simulink model "power_WITHOUT"  (Simulink 7.4)
settings: Solver=FixedStepDiscrete  SolverMode=SingleTasking  StartTime=0.0  StopTime=1  FixedStep=Ts  MaxStep=Ts*2  RelTol=1e-4  AbsTol=1e-4
PreLoadFcn:
  | Ts=50e-6;
undefined symbols (not defined in the file): D1, Delta
libraries: powerlib x9, powerlib_extras x1
Description:
  | Copyright 2008 The MathWorks(TM), Inc.
settings Model: Creator=hyp01  LastModifiedBy=Bharath  ExtModeTrigMode=oneshot  ExtModeArmWhenConnect=off  ExtModeAutoUpdateStatusClock=off
settings DataIOCC: LimitDataPoints=off  SaveFinalState=on  SaveFormat=StructureWithTime  SaveOutput=off  SaveTime=off  SignalLoggingName=sigsOut
settings OptimizationCC: BooleanDataType=off  InlineInvariantSignals=on  InitFltsAndDblsToZero=on  EfficientMapNaN2IntZero=off
settings DebuggingCC: CheckExecutionContextPreStartOutputMsg=on  CheckExecutionContextRuntimeOutputMsg=on  SignalResolutionControl=TryResolveAllWithWarning  SolverPrmCheckMsg=none  MultiTaskDSMMsg=warning  MultiTaskCondExecSysMsg=none  StrictBusMsg=None
settings HardwareCC: TargetUnknown=on
settings RTWCC: IncludeERTFirstTime=on

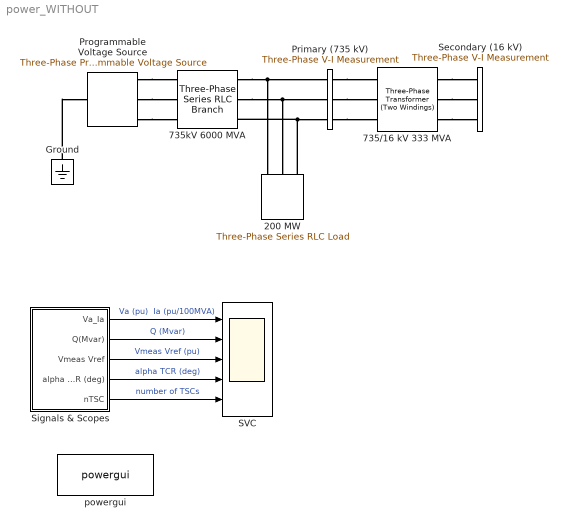
== system power_WITHOUT ==
  200 MW : powerlib/Elements/Three-Phase Series RLC Load  DialogController=POWERSYS.PowerSysDialog  PhysicalDomain=powersysdomain  SubClassName=unknown  LeftPortType=p1  RightPortType=p1  LConnTagsString=A|B|C  Configuration=Y (grounded)  NominalVoltage=735e3  NominalFrequency=60  ActivePower=200e6  InductivePower=0  CapacitivePower=0  Measurements=None
  735/16 kV 333 MVA : powerlib/Elements/Three-Phase Transformer (Two Windings)  DialogController=POWERSYS.PowerSysDialog  SystemSampleTime=-1  Winding1Connection=Yg  UNITS=pu  NominalPower=[333e6 , 60 ]  Winding1=[735e3 , 0.15/30/2 , 0.15*0.7]  Winding2Connection=Delta (D1)  Winding2=[ 16e3 , 0.15/30/2, 0.15*0.3]  SetSaturation=off  Rm=500  Lm=500  Saturation="[ 0,0  ;  0.005,1.2  ;  1.0,1.4 ]"  Hysteresis=off  DataFile='hysteresis'  SetInitialFlux=off  InitialFluxes=[ 0.8 , -0.8 , 0.7 ]  Measurements=None  MoreParameters=off  BreakLoop=off  DataType=off  TransfoNumber=0
  "735kV 6000 MVA " : powerlib/Elements/Three-Phase Series RLC Branch  DialogController=POWERSYS.PowerSysDialog  PhysicalDomain=powersysdomain  SubClassName=unknown  LeftPortType=p1  RightPortType=p1  LConnTagsString=A|B|C  RConnTagsString=A|B|C  BranchType=RL  Resistance=735e3^2/6000e6/10  Inductance=735e3^2/6000e6/(2*pi*60)  Capacitance=1.0  Measurements=None
  Ground : powerlib/Elements/Ground  DialogController=POWERSYS.PowerSysDialog  PhysicalDomain=powersysdomain  SubClassName=unknown  LeftPortType=p1  RightPortType=p1  LConnTagsString=a
  Primary (735 kV) : powerlib/Measurements/Three-Phase V-I Measurement  DialogController=POWERSYS.PowerSysDialog  SystemSampleTime=-1  VoltageMeasurement=phase-to-ground  SetLabelV=on  LabelV=Vabc_Prim  Vpu=on  CurrentMeasurement=yes  SetLabelI=on  LabelI=Iabc_Prim  Ipu=on  Pbase=100e6  Vbase=735e3  OutputType=Magnitude  PhasorSimulation=off  PSBequivalent=0
  Programmable Voltage Source : powerlib/Electrical Sources/Three-Phase Programmable Voltage Source  DialogController=POWERSYS.PowerSysDialog  SystemSampleTime=-1  PositiveSequence="[1.004*735e3 0  60]"  VariationEntity=Amplitude  VariationType=Table of time-amplitude pairs  VariationStep=-0.3  VariationRate=0.5  VariationMagnitude=0.4  VariationFrequency=2  VariationTiming=[0.1 1.2]  VariationPhaseA=off  Amplitudes=[1.0 1.025 0.93 1.0 ]  TimeValues=[0 0.1 0.4 0.7]  HarmonicGeneration=off  HarmonicA=[3 0.2 -25 0]  HarmonicB="[2 0.15  35 2]"  Timing="[0.1  0.6]"
  SVC : Scope  NumInputPorts=5
      settings: YMin=-1.5~-0.7~-1~-1~-1  YMax=1.5~-0.57~1~1~1  SaveName=VIabc_Prim  SampleInput=on  SampleTime=Ts
  Secondary (16 kV) : powerlib/Measurements/Three-Phase V-I Measurement  DialogController=POWERSYS.PowerSysDialog  SystemSampleTime=-1  VoltageMeasurement=phase-to-phase  SetLabelV=on  LabelV=Vabc_Sec  Vpu=on  CurrentMeasurement=no  SetLabelI=off  LabelI=Iabc_Sec  Ipu=off  Pbase=100e6  Vbase=16e3  OutputType=Magnitude  PhasorSimulation=off  PSBequivalent=0
  Signals & Scopes : Subsystem
  powergui : powerlib/powergui  Priority=2  SystemSampleTime=-1  SimulationMode=Discrete  SampleTime=Ts  frequency=60  SPID=off  DisableSnubberDevices=off  DisableRonSwitches=off  DisableVfSwitches=off  SwTol=0  Interpol=off  frequencyindice=60  echomessages=off  HookPort=off  DisplayEquations=off  FunctionMessages=off  EnableUseOfTLC=off  x0status=blocks  RestoreLinks=warning  Frange=[0:2:500]  Ylog=off  Xlog=on  ShowGrid=off  save=off  variable=ZData  ZoomFFT=on  StartTime=0.0  cycles=1  DisplayStyle=1  fundamental=60  FreqAxis=off  MaxFrequency=1000  frequencyindicesteady=1  RmsSteady=2  display=off  Ts=0  methode=off
  wires:
  Signals & Scopes/1(Va_Ia) -> SVC/1  "Va (pu)  Ia (pu/100MVA)"
  Signals & Scopes/3("Vmeas Vref ") -> SVC/3  "Vmeas Vref (pu)"
  Signals & Scopes/5(nTSC) -> SVC/5  "number of TSCs"
  Signals & Scopes/2(Q(Mvar)) -> SVC/2  "Q (Mvar)"
  Signals & Scopes/4(alpha TCR (deg)) -> SVC/4  "alpha TCR (deg)"
  connections:
  Ground/LConn1 -- Programmable Voltage Source/LConn1
  "735kV 6000 MVA "/RConn1 -- Primary (735 kV)/LConn1 -- 200 MW/LConn1
  "735kV 6000 MVA "/RConn2 -- Primary (735 kV)/LConn2 -- 200 MW/LConn2
  735/16 kV 333 MVA/RConn1 -- Secondary (16 kV)/LConn1
  735/16 kV 333 MVA/RConn3 -- Secondary (16 kV)/LConn3
  Programmable Voltage Source/RConn2 -- "735kV 6000 MVA "/LConn2
  Programmable Voltage Source/RConn3 -- "735kV 6000 MVA "/LConn3
  Programmable Voltage Source/RConn1 -- "735kV 6000 MVA "/LConn1
  735/16 kV 333 MVA/RConn2 -- Secondary (16 kV)/LConn2
  200 MW/LConn3 -- "735kV 6000 MVA "/RConn3 -- Primary (735 kV)/LConn3
  Primary (735 kV)/RConn1 -- 735/16 kV 333 MVA/LConn1
  Primary (735 kV)/RConn2 -- 735/16 kV 333 MVA/LConn2
  Primary (735 kV)/RConn3 -- 735/16 kV 333 MVA/LConn3

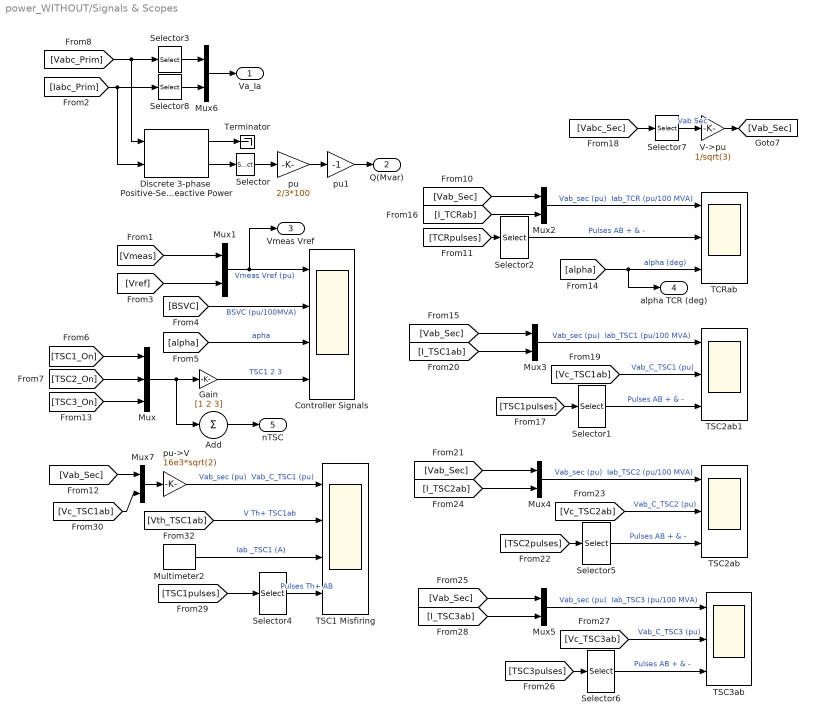
== system power_WITHOUT/Signals & Scopes ==
  Add : Sum  Inputs=+  OutDataType=sfix(16)  OutScaling=2^-10
  Controller Signals : Scope  NumInputPorts=4
      settings: YMin=0.92~-1~90~0  YMax=1.04~2.5~180~3  SaveName=Ctrl_Sig  DataFormat=Array  SampleInput=on  SampleTime=Ts
  Discrete 3-phase  Positive-Sequence  Active & Reactive Power : powerlib_extras/Discrete Measurements/Discrete 3-phase  Positive-Sequence  Active & Reactive Power  DialogController=POWERSYS.PowerSysDialog  SystemSampleTime=-1  Freq=60  Par_Vinit=[1 0]  Par_Iinit=[0.05 90]  Ts=Ts
  Gain : Gain  Gain=[1 2 3]  ParameterDataType=sfix(16)  ParameterScaling=2^0  OutDataType=sfix(16)  OutScaling=2^0  SaturateOnIntegerOverflow=on  OutDataTypeStr=Inherit: Same as input  ParamDataTypeStr=Inherit: Same as input
  Multimeter2 : powerlib/Measurements/Multimeter  Tag=PoWeRsYsTeMmEaSuReMeNt  SystemSampleTime=-1  PhasorSimulation=off  OutputType=Magnitude  sel=1  L=1  Gain=0  yselected={}  PSBOutputType=1  PSBequivalent=0  AxesSetting=[0,0.1,-100,100]  Display=0  SavedBlockNames=-11
      settings: AttributesFormatString=\n
  Mux : Mux  Inputs=3
  Mux{1..7} (7 alike) : Mux  Inputs=2
  Selector : Selector  InputPortWidth=2  IndexOptions=Index vector (dialog)  Indices=2  OutputSizes=1
  Selector{1..2,5..6} (4 alike) : Selector  InputPortWidth=6  IndexOptions=Index vector (dialog)  Indices=[1 2]  OutputSizes=1
  Selector3 : Selector  InputPortWidth=3  IndexOptions=Index vector (dialog)  Indices=1  OutputSizes=1
  Selector4 : Selector  InputPortWidth=6  IndexOptions=Index vector (dialog)  Indices=[1 ]  OutputSizes=1
  Selector7 : Selector  InputPortWidth=3  IndexOptions=Index vector (dialog)  Indices=1  OutputSizes=1
  Selector8 : Selector  InputPortWidth=3  IndexOptions=Index vector (dialog)  Indices=1  OutputSizes=1
  TCRab : Scope  NumInputPorts=3
      settings: TimeRange=0.04  YMin=-1.75~0~97  YMax=1.75~1~108  SaveName=VI_TCRab  SampleInput=on  SampleTime=Ts
  TSC1 Misfiring : Scope  NumInputPorts=4
      settings: TimeRange=0.35  YMin=-30000~-5000~-5000~0  YMax=30000~25000~4000~1  SaveName=VI_TCRab4  SampleInput=on  SampleTime=Ts
  TSC2ab : Scope  NumInputPorts=3
      settings: TimeRange=0.04  YMin=-2~-1.25~0  YMax=2~1.25~1  SaveName=VI_TCRab2  SampleInput=on  SampleTime=Ts
  TSC2ab1 : Scope  NumInputPorts=3
      settings: TimeRange=0.04  YMin=-2~-1.25~0  YMax=2~1.25~1  SaveName=VI_TCRab1  SampleInput=on  SampleTime=Ts
  TSC3ab : Scope  NumInputPorts=3
      settings: TimeRange=0.04  YMin=-2~-1.25~0  YMax=2~1.25~1  SaveName=VI_TCRab3  SampleInput=on  SampleTime=Ts
  Terminator : Terminator
  "V->pu " : Gain  Gain=1/sqrt(3)  ParameterDataType=sfix(16)  ParameterScaling=2^0  OutDataType=sfix(16)  OutScaling=2^0  SaturateOnIntegerOverflow=on  OutDataTypeStr=Inherit: Same as input  ParamDataTypeStr=Inherit: Same as input
  pu : Gain  Gain=2/3*100  ParameterDataType=sfix(16)  ParameterScaling=2^0  OutDataType=sfix(16)  OutScaling=2^0  SaturateOnIntegerOverflow=on  OutDataTypeStr=Inherit: Same as input  ParamDataTypeStr=Inherit: Same as input
  pu->V : Gain  Gain=16e3*sqrt(2)  ParameterDataType=sfix(16)  ParameterScaling=2^0  OutDataType=sfix(16)  OutScaling=2^0  SaturateOnIntegerOverflow=on  OutDataTypeStr=Inherit: Same as input  ParamDataTypeStr=Inherit: Same as input
  pu1 : Gain  Gain=-1  ParameterDataType=sfix(16)  ParameterScaling=2^0  OutDataType=sfix(16)  OutScaling=2^0  SaturateOnIntegerOverflow=on  OutDataTypeStr=Inherit: Same as input  ParamDataTypeStr=Inherit: Same as input
  Va_Ia : Outport  OutDataType=sfix(16)  OutScaling=2^0
  Q(Mvar) : Outport  Port=2  OutDataType=sfix(16)  OutScaling=2^0
  "Vmeas Vref " : Outport  Port=3  OutDataType=sfix(16)  OutScaling=2^0
  alpha TCR (deg) : Outport  Port=4  OutDataType=sfix(16)  OutScaling=2^0
  nTSC : Outport  Port=5  OutDataType=sfix(16)  OutScaling=2^0
  wires:
  [TSC1_On] -> Mux/1
  [TSC2_On] -> Mux/2
  Mux/1 -> Gain/1, Add/1
  [Vmeas] -> Mux1/1
  [Vref] -> Mux1/2
  [Vabc_Prim] -> Discrete 3-phase  Positive-Sequence  Active & Reactive Power/1, Selector3/1
  [Iabc_Prim] -> Discrete 3-phase  Positive-Sequence  Active & Reactive Power/2, Selector8/1
  Discrete 3-phase  Positive-Sequence  Active & Reactive Power/1 -> Terminator/1
  Discrete 3-phase  Positive-Sequence  Active & Reactive Power/2 -> Selector/1
  Selector/1 -> pu/1
  pu/1 -> pu1/1
  [BSVC] -> Controller Signals/2  "BSVC (pu/100MVA)"
  Mux1/1 -> Controller Signals/1, "Vmeas Vref "/1  "Vmeas Vref (pu)"
  [alpha] -> Controller Signals/3  "apha"
  Gain/1 -> Controller Signals/4  "TSC1 2 3"
  [TSC3_On] -> Mux/3
  [TCRpulses] -> Selector2/1
  Selector2/1 -> TCRab/2  "Pulses AB + & -"
  [Vabc_Sec] -> Selector7/1
  Selector7/1 -> "V->pu "/1  "Vab Sec"
  [alpha] -> TCRab/3, alpha TCR (deg)/1  "alpha (deg)"
  [Vab_Sec] -> Mux2/1
  [I_TCRab] -> Mux2/2
  Mux2/1 -> TCRab/1  "Vab_sec (pu)  Iab_TCR (pu/100 MVA)"
  [Vab_Sec] -> Mux3/1
  [I_TSC1ab] -> Mux3/2
  Mux3/1 -> TSC2ab1/1  "Vab_sec (pu)  Iab_TSC1 (pu/100 MVA)"
  [TSC1pulses] -> Selector1/1
  "V->pu "/1 -> [Vab_Sec]
  [Vc_TSC1ab] -> TSC2ab1/2  "Vab_C_TSC1 (pu)"
  [Vab_Sec] -> Mux4/1
  [I_TSC2ab] -> Mux4/2
  Mux4/1 -> TSC2ab/1  "Vab_sec (pu)  Iab_TSC2 (pu/100 MVA)"
  [TSC2pulses] -> Selector5/1
  [Vc_TSC2ab] -> TSC2ab/2  "Vab_C_TSC2 (pu)"
  Selector5/1 -> TSC2ab/3  "Pulses AB + & -"
  [Vab_Sec] -> Mux5/1
  [I_TSC3ab] -> Mux5/2
  Mux5/1 -> TSC3ab/1  "Vab_sec (pu)  Iab_TSC3 (pu/100 MVA)"
  [TSC3pulses] -> Selector6/1
  [Vc_TSC3ab] -> TSC3ab/2  "Vab_C_TSC3 (pu)"
  Selector6/1 -> TSC3ab/3  "Pulses AB + & -"
  pu1/1 -> Q(Mvar)/1
  Add/1 -> nTSC/1
  Selector3/1 -> Mux6/1
  Selector8/1 -> Mux6/2
  Mux6/1 -> Va_Ia/1
  [Vab_Sec] -> Mux7/1
  Mux7/1 -> pu->V/1
  [TSC1pulses] -> Selector4/1
  Selector4/1 -> TSC1 Misfiring/4  "Pulses Th+ AB"
  [Vc_TSC1ab] -> Mux7/2
  Multimeter2/1 -> TSC1 Misfiring/3  "Iab _TSC1 (A)"
  [Vth_TSC1ab] -> TSC1 Misfiring/2  "V Th+ TSC1ab"
  pu->V/1 -> TSC1 Misfiring/1  "Vab_sec (pu)  Vab_C_TSC1 (pu)"
  Selector1/1 -> TSC2ab1/3  "Pulses AB + & -"
